simulink model "pupillary_reflex"  (R2022a)
settings: Solver=VariableStepAuto  StartTime=0.0  StopTime=10.0  RelTol=1e-3
model workspace: external: MATLAB File pupillary_param.m (data not in the file)
values from neighbouring files (symbols this model uses):
  D = 0.18    [pupillary_param.m]    (also in pupillary_stability.m)
  den = [0.0010000000000000002 0.030000000000000006 0.30000000000000004 1         ]    [pupillary_param.m]    (also in pupillary_stability.m = conv(den,expon_den_pade))
  K = 2    [pupillary_param.m]
  num = 1    [pupillary_param.m]    (also in pupillary_stability.m = conv(num,expon_num_pade))
settings Model: Creator=bigba  LastModifiedBy=bigba

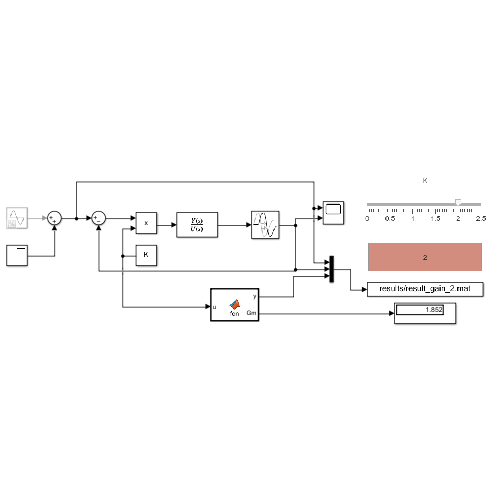
[thumbnail: Simulink's stored preview of the top-level diagram]
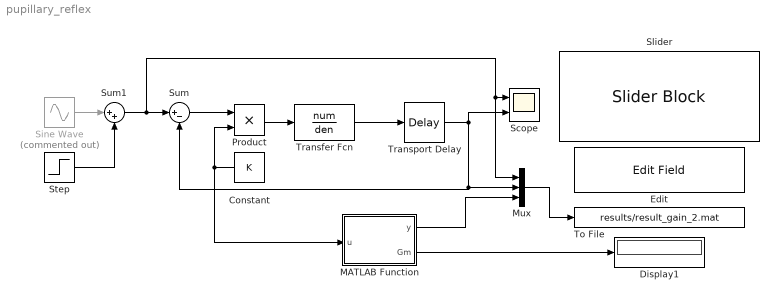
== system pupillary_reflex ==
  Constant : Constant  Value=K
  Display1 : Display
  Edit : EditField  LabelPosition=Hide  ShowInitialText=on  Alignment=Center  Opacity=0.8
  MATLAB Function : MATLAB Function  TreatAsAtomicUnit=on
  Mux : Mux  Inputs=3
  Product : Product
  Scope : Scope  NumInputPorts=2
  Sine Wave : Sin  Commented=on  Frequency=2*pi*0.4  SampleTime=0
  Slider : SliderBlock  ScaleMax=2.5
  Step : Step  SampleTime=0
  Sum : Sum  Inputs=|+-
  Sum1 : Sum  Inputs=|++
  To File : ToFile  InitFcn=|  Filename=results/result_gain_2.mat  SaveFormat=Timeseries
      | wksp=get_param('pupillary_reflex','ModelWorkspace');
      | varValue1 = getVariable(wksp,'K');
      | set_param('pupillary_reflex/To File','FileName',strcat('results/result_gain_',string(varValue1),'.mat'))
  Transfer Fcn : TransferFcn  Numerator=num  Denominator=den
  Transport Delay : TransportDelay  DelayTime=D
  wires:
  Sum1/1 -> Scope/1, Mux/1, Sum/1
  Sum/1 -> Product/1
  Transfer Fcn/1 -> Transport Delay/1
  Transport Delay/1 -> Scope/2, Sum/2, Mux/2
  Product/1 -> Transfer Fcn/1
  Constant/1 -> MATLAB Function/1(u), Product/2
  Mux/1 -> To File/1
  MATLAB Function/1(y) -> Mux/3
  MATLAB Function/2(Gm) -> Display1/1
  Sine Wave/1 -> Sum1/1
  Step/1 -> Sum1/2

== matlab function pupillary_reflex/MATLAB Function ==
  data: u input; y output; Gm output
function [y, Gm] = fcn(u)

coder.extrinsic('set_param')
coder.extrinsic('get_param')
coder.extrinsic('getVariable')
coder.extrinsic('pade')
coder.extrinsic('tf')
coder.extrinsic('margin')



wksp=get_param('pupillary_reflex','ModelWorkspace');
tau = getVariable(wksp,'tau');
D = getVariable(wksp,'D');

% setup color as strings
green='[ 0.2471    0.7804    0.2392]';
red='[0.7255    0.2941    0.2100]';

num_temp=[1];

den_prod=[tau 1];
den_temp=conv(conv(den_prod,den_prod),den_prod);

[expon_num_pade,expon_den_pade]  = pade(D,4);

num=conv(num_temp,expon_num_pade);
den=conv(den_temp,expon_den_pade);

sys=tf(num,den);
Gm_pade=double(0);
Gm_pade=margin(sys);



if u>Gm_pade
    set_param('pupillary_reflex/Edit','BackgroundColor',red);

else
    set_param('pupillary_reflex/Edit','BackgroundColor',green);
end


Gm=Gm_pade;
y = u;
